simulink library "ddm"  (R2021b)
settings: Solver=VariableStepAuto  StartTime=0.0  StopTime=10.0  RelTol=1e-3
undefined symbols (not defined in the file): ADDM_FrTMTqDev_X_Nm, ADDM_RrTMTqDev_X_Nm, ENUM_ADASACCSTA_ERROR, ENUM_ADASACCSTA_OFF, ENUM_ADASACCSTA_STANDBY, ENUM_ALLOWMOV_ALLOWREADY, ENUM_APS, ENUM_BRKSTA_ERROR, ENUM_BRKSTA_OFF, ENUM_BRKSTA_ON, ENUM_BRKSW_INVALID, ENUM_BRKSW_OFF, ENUM_BRKSW_ON, ENUM_CHGPREACTERRSTA_OBCPRE, ENUM_DCDCFAULTSTA_ANYFAULTLV1, ENUM_DCDCFAULTSTA_ANYFAULTLV2, ENUM_DRIVETRAIN_AWD, ENUM_DRIVETRAIN_FWD, ENUM_DRIVETRAIN_RWD, ENUM_EDUDRTSTA_NORMAL, ENUM_EPBERROR_FAILED, ENUM_EPBSTA_APPLIED, ENUM_EPBSTA_RELEASED, ENUM_ESCAPSSta_APSUNAVAILABLE, ENUM_GEARACTUALPOSN_INVALID, ENUM_GEARACTUALPOSN_P, ENUM_HVBATTREADYPRE_READY, ENUM_HWRESETSTA_HWRESETING, ENUM_MCUWARN_LV0, ENUM_MCUWARN_LV1, ENUM_MCUWARN_LV2, ENUM_MCUWARN_LV3, ENUM_MCUWARN_NOERROR, ENUM_OBCFAULTSTA_ANYFAULT, ENUM_PAS_R2F2, ENUM_PDFAULT_BATTPDFAIL, ENUM_PDFAULT_DCDCDISABLE, ENUM_PDFAULT_MCUDISABLE, ENUM_PDFAULT_MCUDISCHRG, ENUM_POWERSTA_OFF, ENUM_POWERSTA_ON, ENUM_POWERSTA_READY, ENUM_POWERSTA_STANDBY, ENUM_PRESSINDI_LOW, ENUM_PUFAULT_BATTUPFAIL, ENUM_PUFAULT_DCDCENABLEFAIL, ENUM_PUFAULT_PRECHRGCHKFAIL, ENUM_PUFAULT_SAFETYCHKFAIL, ENUM_PWRSTASW_OFF, ENUM_PWRSTASW_OFFA, ENUM_PWRSTASW_OFFCHVCHRG, ENUM_PWRSTASW_OFFCLVCHRG, ENUM_PWRSTASW_ON, ENUM_PWRSTASW_ONHVCHRG, ENUM_PWRSTASW_READY, ENUM_PWRSTASW_STANDBY, ENUM_RAPSErrWarnSta_NORMAL, ENUM_RAPSErrWarnSta_RAPSERRLV1, ENUM_SHIFTCOMMAND_P, ENUM_SHIFTERERRSTA_PBUTTONFAILURE ... (+471)
libraries: hcu_lib x540, simulink x3
(part 9 of 26)

== system ddm/DDM/DDM/PMM/Fault level ==
  task_time_s : Inport
  VPMM_PwrStaSW_enum : Inport  Port=2
  VPMM_PowerSta_enum : Inport  Port=3
  VINP_BMSWarn1_flg : Inport  Port=4
  VINP_BMSWarn2_flg : Inport  Port=5
  VINP_BMSWarn3_flg : Inport  Port=6
  VINP_BMSWarn4_flg : Inport  Port=7
  VINP_BMSWarn5_flg : Inport  Port=8
  VINP_BMSWarn6_flg : Inport  Port=9
  VINP_BMSWarn7_flg : Inport  Port=10
  VINP_BMSWarn8_flg : Inport  Port=11
  VINP_DCDCFaultSta_enum : Inport  Port=12
  VPMM_DrivetrainSelect_enum : Inport  Port=13
  VDDM_C3BMS6LCCFS_flg : Inport  Port=14
  VDDM_C3CCU2LCCFS_flg : Inport  Port=15
  VDDM_MCUF1NoComCFS_flg : Inport  Port=16
  VDDM_MCUR1NoComCFS_flg : Inport  Port=17
  VDDM_MCUWarnF_enum : Inport  Port=18
  VDDM_MCUWarnR_enum : Inport  Port=19
  VINP_OBCFaultSta_enum : Inport  Port=20
  DTC_clear_request : Inport  Port=21
  No_CAN3_BUS_OFF : Inport  Port=22
  VDDM_C3CCU2RCCFS_flg : Inport  Port=23
  VDDM_C3CCU2CSCFS_flg : Inport  Port=24
  VDDM_MCUR1RCErrCFS_flg : Inport  Port=25
  VDDM_MCUR1CSErrCFS_flg : Inport  Port=26
  VDDM_MCUF1RCErrCFS_flg : Inport  Port=27
  VDDM_MCUF1CSErrCFS_flg : Inport  Port=28
  VDDM_C3BMS6RCCFS_flg : Inport  Port=29
  VDDM_C3BMS6CSCFS_flg : Inport  Port=30
  No_CAN1_BUS_OFF : Inport  Port=31
  VDDM_ESC1SigErr_flg : Inport  Port=32
  VDDM_ESC5SigErr_flg : Inport  Port=33
  ZoneFrMalfunLevel_enum : Inport  Port=34
  VDDM_FrVCUNoComCFS_flg : Inport  Port=35
  VINP_ShifterFailsta_enum : Inport  Port=36
  VDDM_Shifter1NoComCFS_flg : Inport  Port=37
  VDDM_Shifter1RCErrCFS_flg : Inport  Port=38
  VDDM_Shifter1CSErrCFS_flg : Inport  Port=39
  VINP_ZoneDrMalfunLevel_enum : Inport  Port=40
  No_CAN4_BUS_OFF : Inport  Port=41
  VDDM_DrVCUNoComCFS_flg : Inport  Port=42
  Fault level 1 subsystem error : Subsystem
  Fault level 2 subsystem error : Subsystem
  Fault level 3 subsystem error : Subsystem
  Fault level 4 subsystem error1 : Subsystem
  VDDM_Lv1ErrDTC_raw32 : Outport
  VDDM_Lv2ErrDTC_raw32 : Outport  Port=2
  VDDM_Lv3ErrDTC_raw32 : Outport  Port=3
  VDDM_Lv4ErrDTC_raw32 : Outport  Port=4
  VDDM_Lv1ErrCFS_flg : Outport  Port=5
  VDDM_Lv2ErrCFS_flg : Outport  Port=6
  VDDM_Lv3ErrCFS_flg : Outport  Port=7
  VDDM_Lv4ErrCFS_flg : Outport  Port=8
  VDDM_EDriveSysErrFaultLv1_flg : Outport  Port=9
  wires:
  [No_CAN3_BUS_OFF] -> Fault level 4 subsystem error1/8(No_CAN3_BUS_OFF)
  [DTC_clear_request] -> Fault level 4 subsystem error1/7(DTC_clear_request)
  [DTC_clear_request] -> Fault level 3 subsystem error/11(DTC_clear_request)
  [No_CAN3_BUS_OFF] -> Fault level 3 subsystem error/12(No_CAN3_BUS_OFF)
  [No_CAN3_BUS_OFF] -> Fault level 2 subsystem error/15(No_CAN3_BUS_OFF)
  [DTC_clear_request] -> Fault level 2 subsystem error/14(DTC_clear_request)
  [DTC_clear_request] -> Fault level 1 subsystem error/16(DTC_clear_request)
  [No_CAN3_BUS_OFF] -> Fault level 1 subsystem error/17(No_CAN3_BUS_OFF)
  DTC_clear_request/1 -> [DTC_clear_request]
  No_CAN3_BUS_OFF/1 -> [No_CAN3_BUS_OFF]
  [VDDM_MCUWarnR_enum] -> Fault level 1 subsystem error/13(VDDM_MCUWarnR_enum)
  [VDDM_MCUWarnF_enum] -> Fault level 1 subsystem error/12(VDDM_MCUWarnF_enum)
  [VDDM_MCUWarnF_enum] -> Fault level 3 subsystem error/8(VDDM_MCUWarnF_enum)
  [VDDM_MCUWarnR_enum] -> Fault level 3 subsystem error/9(VDDM_MCUWarnR_enum)
  [VPMM_DrivetrainSelect_enum] -> Fault level 3 subsystem error/10(VPMM_DrivetrainSelect_enum)
  [VDDM_MCUWarnR_enum] -> Fault level 2 subsystem error/12(VDDM_MCUWarnR_enum)
  [VDDM_MCUWarnF_enum] -> Fault level 2 subsystem error/11(VDDM_MCUWarnF_enum)
  [VPMM_DrivetrainSelect_enum] -> Fault level 2 subsystem error/13(VPMM_DrivetrainSelect_enum)
  [VINP_OBCFaultSta_enum] -> Fault level 1 subsystem error/14(VINP_OBCFaultSta_enum)
  VINP_OBCFaultSta_enum/1 -> [VINP_OBCFaultSta_enum]
  VDDM_MCUWarnR_enum/1 -> [VDDM_MCUWarnR_enum]
  VDDM_MCUWarnF_enum/1 -> [VDDM_MCUWarnF_enum]
  [VDDM_C3CCU2LCCFS_flg] -> Fault level 2 subsystem error/5(VDDM_C3CCU2LCCFS_flg)
  [VDDM_C3CCU2LCCFS_flg] -> Fault level 1 subsystem error/5(VDDM_C3CCU2LCCFS_flg)
  VDDM_C3CCU2LCCFS_flg/1 -> [VDDM_C3CCU2LCCFS_flg]
  [VDDM_C3BMS6LCCFS_flg] -> Fault level 4 subsystem error1/4(VDDM_C3BMS6LCCFS_flg)
  [VDDM_C3BMS6LCCFS_flg] -> Fault level 3 subsystem error/4(VDDM_C3BMS6LCCFS_flg)
  [VDDM_MCUR1NoComCFS_flg] -> Fault level 3 subsystem error/6(VDDM_MCUR1NoComCFS_flg)
  [VDDM_MCUF1NoComCFS_flg] -> Fault level 3 subsystem error/5(VDDM_MCUF1NoComCFS_flg)
  [VDDM_MCUF1NoComCFS_flg] -> Fault level 2 subsystem error/6(VDDM_MCUF1NoComCFS_flg)
  [VDDM_MCUR1NoComCFS_flg] -> Fault level 2 subsystem error/7(VDDM_MCUR1NoComCFS_flg)
  [VDDM_MCUF1NoComCFS_flg] -> Fault level 1 subsystem error/6(VDDM_MCUF1NoComCFS_flg)
  [VDDM_MCUR1NoComCFS_flg] -> Fault level 1 subsystem error/7(VDDM_MCUR1NoComCFS_flg)
  VDDM_MCUF1NoComCFS_flg/1 -> [VDDM_MCUF1NoComCFS_flg]
  VDDM_MCUR1NoComCFS_flg/1 -> [VDDM_MCUR1NoComCFS_flg]
  [VDDM_C3BMS6LCCFS_flg] -> Fault level 2 subsystem error/4(VDDM_C3BMS6LCCFS_flg)
  [VDDM_C3BMS6LCCFS_flg] -> Fault level 1 subsystem error/4(VDDM_C3BMS6LCCFS_flg)
  VDDM_C3BMS6LCCFS_flg/1 -> [VDDM_C3BMS6LCCFS_flg]
  [task_time_s] -> Fault level 4 subsystem error1/1(task_time_s)
  [VPMM_DrivetrainSelect_enum] -> Fault level 1 subsystem error/15(VPMM_DrivetrainSelect_enum)
  VPMM_DrivetrainSelect_enum/1 -> [VPMM_DrivetrainSelect_enum]
  [VPMM_PowerSta_enum] -> Fault level 3 subsystem error/2(VPMM_PowerSta_enum)
  [VPMM_PwrStaSW_enum] -> Fault level 3 subsystem error/3(VPMM_PwrStaSW_enum)
  [task_time_s] -> Fault level 3 subsystem error/1(task_time_s)
  [VINP_DCDCFaultSta_enum] -> Fault level 1 subsystem error/11(VINP_DCDCFaultSta_enum)
  [VINP_DCDCFaultSta_enum] -> Fault level 2 subsystem error/10(VINP_DCDCFaultSta_enum)
  VINP_DCDCFaultSta_enum/1 -> [VINP_DCDCFaultSta_enum]
  [task_time_s] -> Fault level 2 subsystem error/1(task_time_s)
  [VPMM_PwrStaSW_enum] -> Fault level 2 subsystem error/3(VPMM_PwrStaSW_enum)
  [VPMM_PowerSta_enum] -> Fault level 2 subsystem error/2(VPMM_PowerSta_enum)
  [VPMM_PowerSta_enum] -> Fault level 1 subsystem error/2(VPMM_PowerSta_enum)
  [VPMM_PwrStaSW_enum] -> Fault level 1 subsystem error/3(VPMM_PwrStaSW_enum)
  [task_time_s] -> Fault level 1 subsystem error/1(task_time_s)
  VPMM_PowerSta_enum/1 -> [VPMM_PowerSta_enum]
  VPMM_PwrStaSW_enum/1 -> [VPMM_PwrStaSW_enum]
  task_time_s/1 -> [task_time_s]
  [VDDM_C3CCU2RCCFS_flg] -> Fault level 1 subsystem error/18(VDDM_C3CCU2RCCFS_flg)
  [VDDM_C3CCU2CSCFS_flg] -> Fault level 1 subsystem error/19(VDDM_C3CCU2CSCFS_flg)
  [VDDM_MCUR1RCErrCFS_flg] -> Fault level 1 subsystem error/20(VDDM_MCUR1RCErrCFS_flg)
  [VDDM_MCUR1CSErrCFS_flg] -> Fault level 1 subsystem error/21(VDDM_MCUR1CSErrCFS_flg)
  [VDDM_MCUF1RCErrCFS_flg] -> Fault level 1 subsystem error/22(VDDM_MCUF1RCErrCFS_flg)
  [VDDM_MCUF1CSErrCFS_flg] -> Fault level 1 subsystem error/23(VDDM_MCUF1CSErrCFS_flg)
  [VDDM_C3BMS6RCCFS_flg] -> Fault level 1 subsystem error/24(VDDM_C3BMS6RCCFS_flg)
  [VDDM_C3BMS6CSCFS_flg] -> Fault level 1 subsystem error/25(VDDM_C3BMS6CSCFS_flg)
  [No_CAN1_BUS_OFF] -> Fault level 1 subsystem error/26(No_CAN1_BUS_OFF)
  [VDDM_ESC1SigErr_flg] -> Fault level 1 subsystem error/27(VDDM_ESC1SigErr_flg)
  [VDDM_ESC5SigErr_flg] -> Fault level 1 subsystem error/28(VDDM_ESC5SigErr_flg)
  [VINP_ShifterFailsta_enum] -> Fault level 1 subsystem error/29(VINP_ShifterFailsta_enum)
  [VDDM_Shifter1NoComCFS_flg] -> Fault level 1 subsystem error/30(VDDM_Shifter1NoComCFS_flg)
  [VDDM_Shifter1RCErrCFS_flg] -> Fault level 1 subsystem error/31(VDDM_Shifter1RCErrCFS_flg)
  [VDDM_Shifter1CSErrCFS_flg] -> Fault level 1 subsystem error/32(VDDM_Shifter1CSErrCFS_flg)
  [VINP_ZoneDrMalfunLevel_enum] -> Fault level 1 subsystem error/33(VINP_ZoneDrMalfunLevel_enum)
  [No_CAN4_BUS_OFF] -> Fault level 1 subsystem error/34(No_CAN4_BUS_OFF)
  [VDDM_DrVCUNoComCFS_flg] -> Fault level 1 subsystem error/35(VDDM_DrVCUNoComCFS_flg)
  [ZoneFrMalfunLevel_enum] -> Fault level 1 subsystem error/36(ZoneFrMalfunLevel_enum)
  [VDDM_FrVCUNoComCFS_flg] -> Fault level 1 subsystem error/37(VDDM_FrVCUNoComCFS_flg)
  [VDDM_C3CCU2RCCFS_flg] -> Fault level 2 subsystem error/16(VDDM_C3CCU2RCCFS_flg)
  [VDDM_C3CCU2CSCFS_flg] -> Fault level 2 subsystem error/17(VDDM_C3CCU2CSCFS_flg)
  [VDDM_MCUR1RCErrCFS_flg] -> Fault level 2 subsystem error/18(VDDM_MCUR1RCErrCFS_flg)
  [VDDM_MCUR1CSErrCFS_flg] -> Fault level 2 subsystem error/19(VDDM_MCUR1CSErrCFS_flg)
  [VDDM_MCUF1RCErrCFS_flg] -> Fault level 2 subsystem error/20(VDDM_MCUF1RCErrCFS_flg)
  [VDDM_MCUF1CSErrCFS_flg] -> Fault level 2 subsystem error/21(VDDM_MCUF1CSErrCFS_flg)
  [VDDM_C3BMS6RCCFS_flg] -> Fault level 2 subsystem error/22(VDDM_C3BMS6RCCFS_flg)
  [VDDM_C3BMS6CSCFS_flg] -> Fault level 2 subsystem error/23(VDDM_C3BMS6CSCFS_flg)
  [VINP_ZoneDrMalfunLevel_enum] -> Fault level 2 subsystem error/24(ZoneDrMalfunLevel_enum)
  [No_CAN4_BUS_OFF] -> Fault level 2 subsystem error/25(No_CAN4_BUS_OFF)
  [VDDM_DrVCUNoComCFS_flg] -> Fault level 2 subsystem error/26(VDDM_DrVCUNoComCFS_flg)
  [ZoneFrMalfunLevel_enum] -> Fault level 2 subsystem error/27(ZoneFrMalfunLevel_enum)
  [VDDM_FrVCUNoComCFS_flg] -> Fault level 2 subsystem error/28(VDDM_FrVCUNoComCFS_flg)
  [VDDM_MCUR1RCErrCFS_flg] -> Fault level 3 subsystem error/13(VDDM_MCUR1RCErrCFS_flg)
  [VDDM_MCUR1CSErrCFS_flg] -> Fault level 3 subsystem error/14(VDDM_MCUR1CSErrCFS_flg)
  [VDDM_MCUF1RCErrCFS_flg] -> Fault level 3 subsystem error/15(VDDM_MCUF1RCErrCFS_flg)
  [VDDM_MCUF1CSErrCFS_flg] -> Fault level 3 subsystem error/16(VDDM_MCUF1CSErrCFS_flg)
  [VDDM_C3BMS6RCCFS_flg] -> Fault level 3 subsystem error/17(VDDM_C3BMS6RCCFS_flg)
  [VDDM_C3BMS6CSCFS_flg] -> Fault level 3 subsystem error/18(VDDM_C3BMS6CSCFS_flg)
  [VINP_ZoneDrMalfunLevel_enum] -> Fault level 3 subsystem error/19(ZoneDrMalfunLevel_enum)
  [No_CAN4_BUS_OFF] -> Fault level 3 subsystem error/20(No_CAN4_BUS_OFF)
  [VDDM_DrVCUNoComCFS_flg] -> Fault level 3 subsystem error/21(VDDM_DrVCUNoComCFS_flg)
  [ZoneFrMalfunLevel_enum] -> Fault level 3 subsystem error/22(ZoneFrMalfunLevel_enum)
  [VDDM_FrVCUNoComCFS_flg] -> Fault level 3 subsystem error/23(VDDM_FrVCUNoComCFS_flg)
  [VPMM_PwrStaSW_enum] -> Fault level 4 subsystem error1/3(VPMM_PwrStaSW_enum)
  [VPMM_PowerSta_enum] -> Fault level 4 subsystem error1/2(VPMM_PowerSta_enum)
  [VDDM_C3BMS6RCCFS_flg] -> Fault level 4 subsystem error1/9(VDDM_C3BMS6RCCFS_flg)
  [VDDM_C3BMS6CSCFS_flg] -> Fault level 4 subsystem error1/10(VDDM_C3BMS6CSCFS_flg)
  [VINP_ZoneDrMalfunLevel_enum] -> Fault level 4 subsystem error1/11(ZoneDrMalfunLevel_enum)
  [No_CAN4_BUS_OFF] -> Fault level 4 subsystem error1/12(No_CAN4_BUS_OFF)
  [VDDM_DrVCUNoComCFS_flg] -> Fault level 4 subsystem error1/13(VDDM_DrVCUNoComCFS_flg)
  [ZoneFrMalfunLevel_enum] -> Fault level 4 subsystem error1/14(ZoneFrMalfunLevel_enum)
  [VDDM_FrVCUNoComCFS_flg] -> Fault level 4 subsystem error1/15(VDDM_FrVCUNoComCFS_flg)
  VINP_BMSWarn1_flg/1 -> [VINP_BMSWarn1_flg]
  VINP_BMSWarn2_flg/1 -> [VINP_BMSWarn2_flg]
  VINP_BMSWarn3_flg/1 -> [VINP_BMSWarn3_flg]
  VINP_BMSWarn4_flg/1 -> [VINP_BMSWarn4_flg]
  VINP_BMSWarn5_flg/1 -> [VINP_BMSWarn5_flg]
  VINP_BMSWarn6_flg/1 -> [VINP_BMSWarn6_flg]
  VINP_BMSWarn7_flg/1 -> [VINP_BMSWarn7_flg]
  VINP_BMSWarn8_flg/1 -> [VINP_BMSWarn8_flg]
  [VINP_BMSWarn1_flg] -> Fault level 1 subsystem error/8(VINP_BMSWarn1_flg)
  [VINP_BMSWarn2_flg] -> Fault level 1 subsystem error/9(VINP_BMSWarn2_flg)
  [VINP_BMSWarn3_flg] -> Fault level 1 subsystem error/10(VINP_BMSWarn3_flg)
  [VINP_BMSWarn4_flg] -> Fault level 2 subsystem error/8(VINP_BMSWarn4_flg)
  [VINP_BMSWarn5_flg] -> Fault level 2 subsystem error/9(VINP_BMSWarn5_flg)
  [VINP_BMSWarn6_flg] -> Fault level 3 subsystem error/7(VINP_BMSWarn6_flg)
  [VINP_BMSWarn7_flg] -> Fault level 4 subsystem error1/5(VINP_BMSWarn7_flg)
  [VINP_BMSWarn8_flg] -> Fault level 4 subsystem error1/6(VINP_BMSWarn8_flg)
  Fault level 1 subsystem error/1(VDDM_Lv1ErrCFS_flg) -> [VDDM_Lv1ErrCFS_flg]
  Fault level 1 subsystem error/2(VDDM_Lv1ErrDTC_raw32) -> [VDDM_Lv1ErrDTC_raw32]
  Fault level 2 subsystem error/1(VDDM_Lv2ErrCFS_flg) -> [VDDM_Lv2ErrCFS_flg]
  Fault level 3 subsystem error/1(VDDM_Lv3ErrCFS_flg) -> [VDDM_Lv3ErrCFS_flg]
  Fault level 4 subsystem error1/1(VDDM_Lv4ErrCFS_flg) -> [VDDM_Lv4ErrCFS_flg]
  Fault level 2 subsystem error/2(VDDM_Lv2ErrDTC_raw32) -> [VDDM_Lv2ErrDTC_raw32]
  Fault level 3 subsystem error/2(VDDM_Lv3ErrDTC_raw32) -> [VDDM_Lv3ErrDTC_raw32]
  Fault level 4 subsystem error1/2(VDDM_Lv4ErrDTC_raw32) -> [VDDM_Lv4ErrDTC_raw32]
  [VDDM_Lv1ErrDTC_raw32] -> VDDM_Lv1ErrDTC_raw32/1
  [VDDM_Lv2ErrDTC_raw32] -> VDDM_Lv2ErrDTC_raw32/1
  [VDDM_Lv3ErrDTC_raw32] -> VDDM_Lv3ErrDTC_raw32/1
  [VDDM_Lv4ErrDTC_raw32] -> VDDM_Lv4ErrDTC_raw32/1
  [VDDM_Lv1ErrCFS_flg] -> VDDM_Lv1ErrCFS_flg/1
  [VDDM_Lv2ErrCFS_flg] -> VDDM_Lv2ErrCFS_flg/1
  [VDDM_Lv3ErrCFS_flg] -> VDDM_Lv3ErrCFS_flg/1
  [VDDM_Lv4ErrCFS_flg] -> VDDM_Lv4ErrCFS_flg/1
  VDDM_MCUF1RCErrCFS_flg/1 -> [VDDM_MCUF1RCErrCFS_flg]
  VDDM_C3BMS6RCCFS_flg/1 -> [VDDM_C3BMS6RCCFS_flg]
  VDDM_MCUR1RCErrCFS_flg/1 -> [VDDM_MCUR1RCErrCFS_flg]
  VDDM_MCUR1CSErrCFS_flg/1 -> [VDDM_MCUR1CSErrCFS_flg]
  VDDM_C3CCU2CSCFS_flg/1 -> [VDDM_C3CCU2CSCFS_flg]
  VDDM_C3CCU2RCCFS_flg/1 -> [VDDM_C3CCU2RCCFS_flg]
  VDDM_MCUF1CSErrCFS_flg/1 -> [VDDM_MCUF1CSErrCFS_flg]
  VDDM_ESC5SigErr_flg/1 -> [VDDM_ESC5SigErr_flg]
  VDDM_ESC1SigErr_flg/1 -> [VDDM_ESC1SigErr_flg]
  No_CAN1_BUS_OFF/1 -> [No_CAN1_BUS_OFF]
  VDDM_C3BMS6CSCFS_flg/1 -> [VDDM_C3BMS6CSCFS_flg]
  ZoneFrMalfunLevel_enum/1 -> [ZoneFrMalfunLevel_enum]
  VDDM_FrVCUNoComCFS_flg/1 -> [VDDM_FrVCUNoComCFS_flg]
  No_CAN4_BUS_OFF/1 -> [No_CAN4_BUS_OFF]
  VINP_ZoneDrMalfunLevel_enum/1 -> [VINP_ZoneDrMalfunLevel_enum]
  VDDM_DrVCUNoComCFS_flg/1 -> [VDDM_DrVCUNoComCFS_flg]
  VDDM_Shifter1NoComCFS_flg/1 -> [VDDM_Shifter1NoComCFS_flg]
  VDDM_Shifter1RCErrCFS_flg/1 -> [VDDM_Shifter1RCErrCFS_flg]
  VINP_ShifterFailsta_enum/1 -> [VINP_ShifterFailsta_enum]
  VDDM_Shifter1CSErrCFS_flg/1 -> [VDDM_Shifter1CSErrCFS_flg]
  Fault level 1 subsystem error/3(VDDM_EDriveSysErrFaultLv1_flg) -> [VDDM_EDriveSysErrFaultLv1_flg]
  [VDDM_EDriveSysErrFaultLv1_flg] -> VDDM_EDriveSysErrFaultLv1_flg/1

== system ddm/DDM/DDM/PMM/Key authentication failed ==
  note: Diagnostics and Fault Handling
  note: Test Pass Criteria
  note: Release Condition After Decision
  note: Test Detection Criteria
  task_time_s : Inport
  VPMM_PowerSta_enum : Inport  Port=2
  VPMM_PwrStaSW_enum : Inport  Port=3
  DTC_clear_request : Inport  Port=4
  VDKC_DKCAuthSta_enum : Inport  Port=5
  VINP_CANMsgValidDKC2_flg : Inport  Port=6
  VINP_CANMsgValidDKC1_flg : Inport  Port=7
  VDDM_ClearZevDTCcmd_flg : Inport  Port=8
  Constant1 : Constant  Value=TRUE
  Constant10 : Constant  Value=ENUM_POWERSTA_STANDBY
  Constant12 : Constant  Value=FALSE
  Constant13 : Constant  Value=KDDM_KeyAuthDTC_cnt
  Constant14 : Constant  Value=KDDM_KeyAuthPassTO_s
  Constant17 : Constant  Value=KDDM_KeyAuthPassTO_s
  Constant18 : Constant  Value=KDDM_KeyAuthDTC_cnt
  Constant2 : Constant  Value=ENUM_PWRSTASW_OFF
  Constant22 : Constant  Value=FALSE
  Constant28 : Constant  Value=ENUM_PWRSTASW_OFF
  Constant30 : Constant  Value=KDDM_KeyAuthDiagnosisOffSW_flg
  Constant31 : Constant  Value=ENUM_POWERSTA_OFF
  Constant6 : Constant  Value=ZERO_INT
  Constant9 : Constant  Value=KDDM_KeyAuthDetTO_s
  DTC_Couter1 : hcu_lib/Basic_Blocks/DTC_Couter
  DTC_Info : hcu_lib/Basic_Blocks/DTC_Info
  Equal1 : RelationalOperator  Operator=~=  OutDataTypeStr=boolean  RndMeth=Simplest
  Equal10 : RelationalOperator  Operator===  OutDataTypeStr=boolean  RndMeth=Simplest
  Equal2 : RelationalOperator  Operator=~=  OutDataTypeStr=boolean  RndMeth=Simplest
  Equal8 : RelationalOperator  OutDataTypeStr=boolean  RndMeth=Simplest
  Equal9 : RelationalOperator  Operator===  OutDataTypeStr=boolean  RndMeth=Simplest
  Logical Operator : Logic  Inputs=3  AllPortsSameDT=off  OutDataTypeStr=boolean
  Logical Operator1 : Logic  Inputs=3  AllPortsSameDT=off  OutDataTypeStr=boolean
  Logical Operator16 : Logic  Operator=OR  Inputs=4  AllPortsSameDT=off  OutDataTypeStr=boolean
  Logical Operator17 : Logic  AllPortsSameDT=off  OutDataTypeStr=boolean
  Logical Operator21 : Logic  Operator=NOT  AllPortsSameDT=off  OutDataTypeStr=boolean
  Relational Operator1 : RelationalOperator  Operator=>  OutDataTypeStr=boolean  RndMeth=Simplest
  Switch1 : Switch  Criteria=u2 ~= 0
  Switch8 : Switch  Criteria=u2 ~= 0
  Switch9 : Switch  Criteria=u2 ~= 0
  Terminator : Terminator
  Test Detection Criteria1 : hcu_lib/Basic_Blocks/Test Detection Criteria
  Timer2 : hcu_lib/Basic_Blocks/Timer
  Unit Delay1 : UnitDelay  SampleTime=-1  HasFrameUpgradeWarning=on
  VDDM_KeyAuthDTC_raw32 : Outport
  VDDM_KeyAuthCFS_flg : Outport  Port=2
  wires:
  [VDDM_KeyAuthCFS_flg] -> VDDM_KeyAuthCFS_flg/1
  [VDDM_KeyAuthPass_flg] -> Logical Operator16/3
  [VPMM_PwrStaSW_enum] -> Equal1/1
  Constant28/1 -> Equal1/2
  Test Detection Criteria1/1 -> [VDDM_KeyAuthDet_flg]  "VDDM_KeyAuthDet_flg"
  [VDKC_DKCAuthSta_enum] -> Switch8/1
  Equal9/1 -> Logical Operator17/1
  Constant10/1 -> Equal10/2
  Constant17/1 -> Equal8/2
  Constant14/1 -> Timer2/4
  Constant22/1 -> Switch9/1
  [VPMM_PowerSta_enum] -> Equal10/1
  [VDDM_KeyAuthCFSRls_flg] -> DTC_Couter1/2
  Constant18/1 -> DTC_Couter1/3
  DTC_Couter1/1 -> [VDDM_KeyAuthCFS_flg]  "VDDM_KeyAuthCFS_flg"
  Relational Operator1/1 -> Terminator/1  "VDDM_KeyAuthDFS_flg"
  Timer2/1 -> Equal8/1
  Switch9/1 -> Test Detection Criteria1/1
  Constant12/1 -> Switch1/3
  Logical Operator21/1 -> Timer2/1
  Equal10/1 -> Logical Operator17/2
  DTC_Couter1/2 -> Relational Operator1/1  "VDDM_KeyAuthDTC_cnt"
  Constant31/1 -> Equal9/2
  Logical Operator17/1 -> Logical Operator16/1
  [VDDM_ClearZevDTCcmd_flg] -> Logical Operator16/2
  [task_time_s] -> Timer2/3
  Constant30/1 -> Logical Operator16/4
  Constant1/1 -> Switch8/3
  [VDDM_KeyAuthCFSRls_flg] -> Switch9/2
  Switch1/1 -> Switch9/3
  [task_time_s] -> Test Detection Criteria1/2
  [VPMM_PowerSta_enum] -> Unit Delay1/1
  Switch8/1 -> Logical Operator21/1, Timer2/2
  Equal8/1 -> [VDDM_KeyAuthPass_flg]  "VDDM_KeyAuthPass_flg"
  Constant6/1 -> Relational Operator1/2
  Unit Delay1/1 -> Equal9/1
  Constant9/1 -> Test Detection Criteria1/4
  [VDDM_KeyAuthDet_flg] -> DTC_Couter1/1
  Logical Operator16/1 -> [VDDM_KeyAuthCFSRls_flg]  "VDDM_KeyAuthCFSRls_flg"
  Constant13/1 -> Test Detection Criteria1/3
  VPMM_PowerSta_enum/1 -> [VPMM_PowerSta_enum]
  VPMM_PwrStaSW_enum/1 -> [VPMM_PwrStaSW_enum]
  task_time_s/1 -> [task_time_s]
  VDKC_DKCAuthSta_enum/1 -> [VDKC_DKCAuthSta_enum]
  DTC_clear_request/1 -> [DTC_clear_request]
  [VDDM_KeyAuthPass_flg] -> DTC_Info/2
  [VDDM_KeyAuthCFS_flg] -> DTC_Info/3
  DTC_Info/1 -> VDDM_KeyAuthDTC_raw32/1  "VDDM_KeyAuthDTC_raw32"
  [VDDM_KeyAuthDet_flg] -> DTC_Info/1
  [VDDM_ClearZevDTCcmd_flg] -> DTC_Info/4
  [VDKC_DKCAuthSta_enum] -> Switch1/1
  VINP_CANMsgValidDKC2_flg/1 -> [VINP_CANMsgValidDKC2_flg]
  VINP_CANMsgValidDKC1_flg/1 -> [VINP_CANMsgValidDKC1_flg]
  Logical Operator/1 -> Switch1/2
  Equal1/1 -> Logical Operator/1
  [VINP_CANMsgValidDKC1_flg] -> Logical Operator/2
  [VINP_CANMsgValidDKC2_flg] -> Logical Operator/3
  [VINP_CANMsgValidDKC1_flg] -> Logical Operator1/2
  Equal2/1 -> Logical Operator1/1
  [VPMM_PwrStaSW_enum] -> Equal2/1
  Logical Operator1/1 -> Switch8/2
  Constant2/1 -> Equal2/2
  [VINP_CANMsgValidDKC2_flg] -> Logical Operator1/3
  VDDM_ClearZevDTCcmd_flg/1 -> [VDDM_ClearZevDTCcmd_flg]

== system ddm/DDM/DDM/PMM/LV ==
  task_time_s : Inport
  VPMM_PwrStaSW_enum : Inport  Port=2
  VPMM_PowerSta_enum : Inport  Port=3
  VINP_LVBattDet12V_V : Inport  Port=4
  VINP_CANMsgValidBMS5_flg : Inport  Port=5
  DTC_clear_request : Inport  Port=6
  VDDM_AuxBattVolV_V : Inport  Port=7
  VDDM_ClearZevDTCcmd_flg : Inport  Port=8
  VINP_VehicleType_enum : Inport  Port=9
  Constant1 : Constant  Value=ENUM_VEHICLETYPE_D31L24
  Constant2 : Constant  Value=TRUE
  Constant7 : Constant  Value=ENUM_VEHICLETYPE_D31L24
  Initial LV battery voltage too low : Subsystem
  LV analog input error : Subsystem
  LV power supply voltage too high : Subsystem
  LV power supply voltage too low : Subsystem
  Logical Operator : Logic  Operator=OR  Inputs=4  AllPortsSameDT=off  OutDataTypeStr=boolean
  Logical Operator1 : Logic  Operator=OR  AllPortsSameDT=off  OutDataTypeStr=boolean
  Relational Operator1 : RelationalOperator  Operator=~=  OutDataTypeStr=boolean  RndMeth=Simplest
  Relational Operator5 : RelationalOperator  Operator=~=  OutDataTypeStr=boolean  RndMeth=Simplest
  Switch : Switch  Criteria=u2 ~= 0
  Switch2 : Switch  Criteria=u2 ~= 0
  VDDM_IniLVLoDTC_raw32 : Outport
  VDDM_LVSupLoDTC_raw32 : Outport  Port=2
  VDDM_LVSupHiDTC_raw32 : Outport  Port=3
  VDDM_LVInErrDTC_raw32 : Outport  Port=4
  VDDM_IniLVLoCFS_flg : Outport  Port=5
  VDDM_LVSupLoCFS_flg : Outport  Port=6
  VDDM_LVSupHiCFS_flg : Outport  Port=7
  VDDM_LVInErrCFS_flg : Outport  Port=8
  VDDM_PMMBattErr_flg : Outport  Port=9
  VDDM_EDriveSysErrLVSup_flg : Outport  Port=10
  wires:
  DTC_clear_request/1 -> [DTC_clear_request]
  [VDDM_ClearZevDTCcmd_flg] -> LV power supply voltage too high/6(DTC_clear_request)
  [VDDM_AuxBatVolt_V] -> LV power supply voltage too high/4(VDDM_AuxBatVolt_V)
  [VPMM_PowerSta_enum] -> LV power supply voltage too high/2(VPMM_PowerSta_enum)
  [VINP_CANMsgValidBMS5_flg] -> LV power supply voltage too high/5(VINP_CANMsgValidBMS5_flg)
  [VPMM_PwrStaSW_enum] -> LV power supply voltage too high/3(VPMM_PwrStaSW_enum)
  [task_time_s] -> LV power supply voltage too high/1(task_time_s)
  [VDDM_AuxBatVolt_V] -> LV power supply voltage too low/4(VDDM_AuxBatVolt_V)
  [VINP_CANMsgValidBMS5_flg] -> LV power supply voltage too low/5(VINP_CANMsgValidBMS5_flg)
  [task_time_s] -> LV power supply voltage too low/1(task_time_s)
  [VDDM_ClearZevDTCcmd_flg] -> LV power supply voltage too low/6(DTC_clear_request)
  [VPMM_PwrStaSW_enum] -> LV power supply voltage too low/3(VPMM_PwrStaSW_enum)
  [VPMM_PowerSta_enum] -> LV power supply voltage too low/2(VPMM_PowerSta_enum)
  VINP_LVBattDet12V_V/1 -> [VINP_LVBattDet12V_V]
  task_time_s/1 -> [task_time_s]
  VPMM_PwrStaSW_enum/1 -> [VPMM_PwrStaSW_enum]
  VPMM_PowerSta_enum/1 -> [VPMM_PowerSta_enum]
  LV power supply voltage too low/1(VDDM_LVSupLoDTC_raw32) -> VDDM_LVSupLoDTC_raw32/1  "VDDM_LVSupLoDTC_raw32"
  LV power supply voltage too high/1(VDDM_LVSupHiDTC_raw32) -> VDDM_LVSupHiDTC_raw32/1  "VDDM_LVSupHiDTC_raw32"
  LV power supply voltage too low/2(VDDM_LVSupLoCFS_flg) -> [VDDM_LVSupLoCFS_flg]
  LV power supply voltage too high/2(VDDM_LVSupHiCFS_flg) -> [VDDM_LVSupHiCFS_flg]
  [VPMM_PowerSta_enum] -> LV analog input error/2(VPMM_PowerSta_enum)
  LV analog input error/2(VDDM_LVInErrCFS_flg) -> [VDDM_LVInErrCFS_flg]
  [VDDM_AuxBattVolV_V] -> LV analog input error/6(VDDM_AuxBattVolV_V)
  [VINP_LVBattDet12V_V] -> LV analog input error/3(VINP_LVBattDet12V_V)
  [task_time_s] -> LV analog input error/1(task_time_s)
  [DTC_clear_request] -> LV analog input error/5(DTC_clear_request)
  [VINP_CANMsgValidBMS5_flg] -> LV analog input error/4(VINP_CANMsgValidBMS5_flg)
  LV analog input error/1(VDDM_LVInErrDTC_raw32) -> VDDM_LVInErrDTC_raw32/1
  [VDDM_IniLVLoCFS_flg] -> VDDM_IniLVLoCFS_flg/1
  [VDDM_LVSupLoCFS_flg] -> VDDM_LVSupLoCFS_flg/1
  [VDDM_LVSupHiCFS_flg] -> VDDM_LVSupHiCFS_flg/1
  [VDDM_LVInErrCFS_flg] -> VDDM_LVInErrCFS_flg/1
  VDDM_AuxBattVolV_V/1 -> [VDDM_AuxBattVolV_V]
  [VDDM_IniLVLoCFS_flg] -> Logical Operator/1
  [VDDM_LVSupLoCFS_flg] -> Logical Operator/2
  [VDDM_LVSupHiCFS_flg] -> Logical Operator/3
  [VDDM_LVInErrCFS_flg] -> Logical Operator/4
  Logical Operator/1 -> VDDM_PMMBattErr_flg/1  "VDDM_PMMBattErr_flg"
  VDDM_ClearZevDTCcmd_flg/1 -> [VDDM_ClearZevDTCcmd_flg]
  [VDDM_LVSupLoCFS_flg] -> Logical Operator1/1
  [VDDM_LVSupHiCFS_flg] -> Logical Operator1/2
  Logical Operator1/1 -> VDDM_EDriveSysErrLVSup_flg/1  "VDDM_EDriveSysErrLVSup_flg"
  Switch/1 -> [VDDM_AuxBatVolt_V]  "VDDM_AuxBatVolt_V"
  [VINP_VehicleType_enum] -> Relational Operator5/1
  [VINP_LVBattDet12V_V] -> Switch/3
  Relational Operator5/1 -> Switch/2
  Constant7/1 -> Relational Operator5/2
  [VDDM_AuxBattVolV_V] -> Switch/1
  VINP_VehicleType_enum/1 -> [VINP_VehicleType_enum]
  [VINP_CANMsgValidBMS5_flg] -> Initial LV battery voltage too low/5(VINP_CANMsgValidBMS5_flg)
  [VPMM_PowerSta_enum] -> Initial LV battery voltage too low/2(VPMM_PowerSta_enum)
  Initial LV battery voltage too low/2(VDDM_IniLVLoCFS_flg) -> [VDDM_IniLVLoCFS_flg]
  [VDDM_AuxBatVolt_V] -> Initial LV battery voltage too low/4(VDDM_AuxBatVolt_V)
  Initial LV battery voltage too low/1(VDDM_IniLVLoDTC_raw32) -> VDDM_IniLVLoDTC_raw32/1  "VDDM_IniLVLoDTC_raw32"
  [VDDM_ClearZevDTCcmd_flg] -> Initial LV battery voltage too low/6(DTC_clear_request)
  [task_time_s] -> Initial LV battery voltage too low/1(task_time_s)
  [VPMM_PwrStaSW_enum] -> Initial LV battery voltage too low/3(VPMM_PwrStaSW_enum)
  Switch2/1 -> [VINP_CANMsgValidBMS5_flg]
  Constant1/1 -> Relational Operator1/2
  Relational Operator1/1 -> Switch2/2
  [VINP_VehicleType_enum] -> Relational Operator1/1
  VINP_CANMsgValidBMS5_flg/1 -> Switch2/3
  Constant2/1 -> Switch2/1
  [VINP_VehicleType_enum] -> LV analog input error/7(VINP_VehicleType_enum)

== system ddm/DDM/DDM/PMM/SW failure ==
  task_time_s : Inport
  VPMM_PwrStaSW_enum : Inport  Port=2
  VPMM_PowerSta_enum : Inport  Port=3
  DTC_clear_request : Inport  Port=4
  VINP_DrStSW : Inport  Port=5
  VINP_FLAJARSW : Inport  Port=6
  VINP_FRAJARSW : Inport  Port=7
  VINP_RLAJARSW : Inport  Port=8
  VINP_RRAJARSW : Inport  Port=9
  VINP_HoodSW : Inport  Port=10
  VINP_TailgaSW : Inport  Port=11
  VDDM_ClearZevDTCcmd_flg : Inport  Port=12
  Driver seat switch failure : Subsystem
  FL Door switch failure : Subsystem
  FR Door switch failure : Subsystem
  Hood switch failure : Subsystem
  Logical Operator14 : Logic  Operator=OR  Inputs=6  AllPortsSameDT=off  OutDataTypeStr=boolean
  RL Door switch failure : Subsystem
  RR Door switch failure : Subsystem
  Tailgate switch failure : Subsystem
  VDDM_DrStSWDTC_raw32 : Outport
  VDDM_FLDoorSWDTC_raw32 : Outport  Port=2
  VDDM_RLDoorSWDTC_raw32 : Outport  Port=3
  VDDM_FRDoorSWDTC_raw32 : Outport  Port=4
  VDDM_RRDoorSWDTC_raw32 : Outport  Port=5
  VDDM_HoodSWDTC_raw32 : Outport  Port=6
  VDDM_TailgaSWDTC_raw32 : Outport  Port=7
  VDDM_VCUFLDoorSta_flg : Outport  Port=8
  VDDM_VCUFRDoorSta_flg : Outport  Port=9
  VDDM_VCURLDoorSta_flg : Outport  Port=10
  VDDM_VCURRDoorSta_flg : Outport  Port=11
  VDDM_VCUHoodSWSta_flg : Outport  Port=12
  VDDM_VCUTailgateSWSta_flg : Outport  Port=13
  VDDM_DrStSWCFS_flg : Outport  Port=14
  VDDM_FLDoorSWCFS_flg : Outport  Port=15
  VDDM_RLDoorSWCFS_flg : Outport  Port=16
  VDDM_FRDoorSWCFS_flg : Outport  Port=17
  VDDM_RRDoorSWCFS_flg : Outport  Port=18
  VDDM_HoodSWCFS_flg : Outport  Port=19
  VDDM_TailgaSWCFS_flg : Outport  Port=20
  VDDM_4D2CErr_flg : Outport  Port=21
  wires:
  Tailgate switch failure/2(VDDM_VCUTailgateSWSta_flg) -> VDDM_VCUTailgateSWSta_flg/1
  Tailgate switch failure/1(VDDM_TailgaSWDTC_raw32) -> VDDM_TailgaSWDTC_raw32/1
  [VINP_TailgaSW] -> Tailgate switch failure/4(VINP_TailgaSW)
  [DTC_clear_request] -> Tailgate switch failure/5(DTC_clear_request)
  [VPMM_PwrStaSW_enum] -> Tailgate switch failure/3(VPMM_PwrStaSW_enum)
  [VPMM_PowerSta_enum] -> Tailgate switch failure/2(VPMM_PowerSta_enum)
  [task_time_s] -> Tailgate switch failure/1(task_time_s)
  Hood switch failure/2(VDDM_VCUHoodSWSta_flg) -> VDDM_VCUHoodSWSta_flg/1
  Hood switch failure/1(VDDM_HoodSWDTC_raw32) -> VDDM_HoodSWDTC_raw32/1
  [VDDM_ClearZevDTCcmd_flg] -> Hood switch failure/5(DTC_clear_request)
  [VINP_HoodSW] -> Hood switch failure/4(VINP_HoodSW)
  VINP_TailgaSW/1 -> [VINP_TailgaSW]
  VINP_HoodSW/1 -> [VINP_HoodSW]
  [VPMM_PwrStaSW_enum] -> Hood switch failure/3(VPMM_PwrStaSW_enum)
  [VPMM_PowerSta_enum] -> Hood switch failure/2(VPMM_PowerSta_enum)
  [task_time_s] -> Hood switch failure/1(task_time_s)
  RR Door switch failure/2(VDDM_VCURRDoorSta_flg) -> VDDM_VCURRDoorSta_flg/1
  RR Door switch failure/1(VDDM_RRDoorSWDTC_raw32) -> VDDM_RRDoorSWDTC_raw32/1
  [VDDM_ClearZevDTCcmd_flg] -> RR Door switch failure/5(DTC_clear_request)
  [VINP_RRAJARSW] -> RR Door switch failure/4(VINP_RRAJARSW)
  [VPMM_PwrStaSW_enum] -> RR Door switch failure/3(VPMM_PwrStaSW_enum)
  [VPMM_PowerSta_enum] -> RR Door switch failure/2(VPMM_PowerSta_enum)
  [task_time_s] -> RR Door switch failure/1(task_time_s)
  RL Door switch failure/2(VDDM_VCURLDoorSta_flg) -> VDDM_VCURLDoorSta_flg/1
  RL Door switch failure/1(VDDM_RLDoorSWDTC_raw32) -> VDDM_RLDoorSWDTC_raw32/1
  [VDDM_ClearZevDTCcmd_flg] -> RL Door switch failure/5(DTC_clear_request)
  [VINP_RLAJARSW] -> RL Door switch failure/4(VINP_RLAJARSW)
  [task_time_s] -> RL Door switch failure/1(task_time_s)
  [VPMM_PowerSta_enum] -> RL Door switch failure/2(VPMM_PowerSta_enum)
  [VPMM_PwrStaSW_enum] -> RL Door switch failure/3(VPMM_PwrStaSW_enum)
  FR Door switch failure/2(VDDM_VCUFRDoorSta_flg) -> VDDM_VCUFRDoorSta_flg/1
  FR Door switch failure/1(VDDM_FRDoorSWDTC_raw32) -> VDDM_FRDoorSWDTC_raw32/1
  [VDDM_ClearZevDTCcmd_flg] -> FR Door switch failure/5(DTC_clear_request)
  [VINP_FRAJARSW] -> FR Door switch failure/4(VINP_FRAJARSW)
  [VPMM_PwrStaSW_enum] -> FR Door switch failure/3(VPMM_PwrStaSW_enum)
  [VPMM_PowerSta_enum] -> FR Door switch failure/2(VPMM_PowerSta_enum)
  [task_time_s] -> FR Door switch failure/1(task_time_s)
  FL Door switch failure/2(VDDM_VCUFLDoorSta_flg) -> VDDM_VCUFLDoorSta_flg/1
  FL Door switch failure/1(VDDM_FLDoorSWDTC_raw32) -> VDDM_FLDoorSWDTC_raw32/1
  [VDDM_ClearZevDTCcmd_flg] -> FL Door switch failure/5(DTC_clear_request)
  [VINP_FLAJARSW] -> FL Door switch failure/4(VINP_FLAJARSW)
  [VPMM_PwrStaSW_enum] -> FL Door switch failure/3(VPMM_PwrStaSW_enum)
  [VPMM_PowerSta_enum] -> FL Door switch failure/2(VPMM_PowerSta_enum)
  [task_time_s] -> FL Door switch failure/1(task_time_s)
  VINP_RRAJARSW/1 -> [VINP_RRAJARSW]
  VINP_RLAJARSW/1 -> [VINP_RLAJARSW]
  VINP_FRAJARSW/1 -> [VINP_FRAJARSW]
  VINP_FLAJARSW/1 -> [VINP_FLAJARSW]
  Driver seat switch failure/2(VDDM_DrStSWCFS_flg) -> VDDM_DrStSWCFS_flg/1
  DTC_clear_request/1 -> [DTC_clear_request]
  VPMM_PowerSta_enum/1 -> [VPMM_PowerSta_enum]
  VPMM_PwrStaSW_enum/1 -> [VPMM_PwrStaSW_enum]
  task_time_s/1 -> [task_time_s]
  VINP_DrStSW/1 -> [VINP_DrStSW]
  [task_time_s] -> Driver seat switch failure/1(task_time_s)
  [VINP_DrStSW] -> Driver seat switch failure/4(VINP_DrStSW)
  [VDDM_ClearZevDTCcmd_flg] -> Driver seat switch failure/5(DTC_clear_request)
  [VPMM_PwrStaSW_enum] -> Driver seat switch failure/3(VPMM_PwrStaSW_enum)
  [VPMM_PowerSta_enum] -> Driver seat switch failure/2(VPMM_PowerSta_enum)
  Driver seat switch failure/1(VDDM_DrStSWDTC_raw32) -> VDDM_DrStSWDTC_raw32/1
  FL Door switch failure/3(VDDM_FLDoorSWCFS_flg) -> [VDDM_FLDoorSWCFS_flg], VDDM_FLDoorSWCFS_flg/1
  RL Door switch failure/3(VDDM_RLDoorSWCFS_flg) -> [VDDM_RLDoorSWCFS_flg], VDDM_RLDoorSWCFS_flg/1
  FR Door switch failure/3(VDDM_FRDoorSWCFS_flg) -> [VDDM_FRDoorSWCFS_flg], VDDM_FRDoorSWCFS_flg/1
  RR Door switch failure/3(VDDM_RRDoorSWCFS_flg) -> [VDDM_RRDoorSWCFS_flg], VDDM_RRDoorSWCFS_flg/1
  Hood switch failure/3(VDDM_HoodSWCFS_flg) -> [VDDM_HoodSWCFS_flg], VDDM_HoodSWCFS_flg/1
  Tailgate switch failure/3(VDDM_TailgaSWCFS_flg) -> [VDDM_TailgaSWCFS_flg], VDDM_TailgaSWCFS_flg/1
  VDDM_ClearZevDTCcmd_flg/1 -> [VDDM_ClearZevDTCcmd_flg]
  [VDDM_RLDoorSWCFS_flg] -> Logical Operator14/3
  [VDDM_TailgaSWCFS_flg] -> Logical Operator14/6
  [VDDM_FLDoorSWCFS_flg] -> Logical Operator14/1
  [VDDM_HoodSWCFS_flg] -> Logical Operator14/5
  [VDDM_RRDoorSWCFS_flg] -> Logical Operator14/4
  [VDDM_FRDoorSWCFS_flg] -> Logical Operator14/2
  Logical Operator14/1 -> [VDDM_4D2CErr_flg]  "VDDM_4D2CErr_flg"
  [VDDM_4D2CErr_flg] -> VDDM_4D2CErr_flg/1

== system ddm/DDM/DDM/PMM/System conditions of ON to READY not satisfied ==
  note: Release Condition After Decision
  note: Test Detection Criteria
  note: Diagnostics and Fault Handling
  note: Test Pass Criteria
  task_time_s : Inport
  VPMM_PowerSta_enum : Inport  Port=2
  VPMM_PwrStaSW_enum : Inport  Port=3
  DTC_clear_request : Inport  Port=4
  VPMM_MCUReady_flg : Inport  Port=5
  VINP_AllowMovThd_OTA_enum : Inport  Port=6
  VDDM_KeyAuthCFS_flg : Inport  Port=7
  VDDM_FLDoorSWCFS_flg : Inport  Port=8
  VDDM_RLDoorSWCFS_flg : Inport  Port=9
  VDDM_FRDoorSWCFS_flg : Inport  Port=10
  VDDM_RRDoorSWCFS_flg : Inport  Port=11
  VDDM_HoodSWCFS_flg : Inport  Port=12
  VDDM_TailgaSWCFS_flg : Inport  Port=13
  Constant{1..2,12,22} (4 alike) : Constant  Value=FALSE
  Constant10 : Constant  Value=ENUM_POWERSTA_STANDBY
  Constant13 : Constant  Value=KDDM_ONtoRdyPassTO_s
  Constant14 : Constant  Value=KDDM_ONtoRdyPassTO_s
  Constant17 : Constant  Value=KDDM_ONtoRdyDetTO_s
  Constant18 : Constant  Value=KDDM_ONtoRdyDTC_cnt
  Constant28 : Constant  Value=ENUM_PWRSTASW_ON
  Constant29 : Constant  Value=ENUM_PWRSTASW_ON
  Constant3 : Constant  Value=TRUE
  Constant30 : Constant  Value=KDDM_ONtoRdyDiagnosisOffSW_flg
  Constant31 : Constant  Value=ENUM_POWERSTA_OFF
  Constant32 : Constant  Value=ENUM_ALLOWMOV_ALLOWREADY
  Constant34 : Constant  Value=ZERO_INT
  Constant35 : Constant  Value=KDDM_ONtoRdyDTC_cnt
  Constant4 : Constant  Value=TRUE
  Constant5 : Constant  Value=ENUM_ALLOWMOV_ALLOWREADY
  Constant6 : Constant  Value=TRUE
  DTC_Couter1 : hcu_lib/Basic_Blocks/DTC_Couter
  DTC_Info : hcu_lib/Basic_Blocks/DTC_Info
  Equal1 : RelationalOperator  Operator=~=  OutDataTypeStr=boolean  RndMeth=Simplest
  Equal{8,10,12,14} (4 alike) : RelationalOperator  Operator===  OutDataTypeStr=boolean  RndMeth=Simplest
  Equal11 : RelationalOperator  Operator=~=  OutDataTypeStr=boolean  RndMeth=Simplest
  Equal13 : RelationalOperator  OutDataTypeStr=boolean  RndMeth=Simplest
  Logical Operator1 : Logic  Operator=NOT  AllPortsSameDT=off  OutDataTypeStr=boolean
  Logical Operator14 : Logic  Operator=NOT  AllPortsSameDT=off  OutDataTypeStr=boolean
  Logical Operator16 : Logic  Operator=OR  Inputs=4  AllPortsSameDT=off  OutDataTypeStr=boolean
  Logical Operator17 : Logic  AllPortsSameDT=off  OutDataTypeStr=boolean
  Logical Operator2 : Logic  Operator=OR  Inputs=9  AllPortsSameDT=off  OutDataTypeStr=boolean
  Logical Operator20 : Logic  Operator=OR  Inputs=9  AllPortsSameDT=off  OutDataTypeStr=boolean
  Logical Operator21 : Logic  Operator=NOT  AllPortsSameDT=off  OutDataTypeStr=boolean
  Relational Operator1 : RelationalOperator  Operator=>  OutDataTypeStr=boolean  RndMeth=Simplest
  Switch{1..4,9} (5 alike) : Switch  Criteria=u2 ~= 0
  Terminator : Terminator
  Test Detection Criteria1 : hcu_lib/Basic_Blocks/Test Detection Criteria
  Timer2 : hcu_lib/Basic_Blocks/Timer
  Unit Delay1 : UnitDelay  SampleTime=-1  HasFrameUpgradeWarning=on
  VDDM_ONtoRdyDTC_raw32 : Outport
  VDDM_ONtoRdyCFS_flg : Outport  Port=2
  VDDM_EDriveSysErrONtoRdy_flg : Outport  Port=3
  VDDM_SysAllowReadySta_flg : Outport  Port=4
  wires:
  [VDDM_RRDoorSWCFS_flg] -> Logical Operator2/7
  Logical Operator2/1 -> Switch3/1
  [VDDM_FRDoorSWCFS_flg] -> Logical Operator2/6
  [VDDM_RLDoorSWCFS_flg] -> Logical Operator2/5
  [VDDM_FLDoorSWCFS_flg] -> Logical Operator2/4
  [VPMM_MCUReady_flg] -> Logical Operator1/1
  [VDDM_TailgaSWCFS_flg] -> Logical Operator2/9
  [VDDM_HoodSWCFS_flg] -> Logical Operator2/8
  [VDDM_KeyAuthCFS_flg] -> Logical Operator2/3
  Equal1/1 -> Logical Operator2/2
  Constant5/1 -> Equal1/2
  [VINP_AllowMovThd_OTA_enum] -> Equal1/1
  Logical Operator1/1 -> Logical Operator2/1
  [VDDM_TailgaSWCFS_flg] -> Logical Operator20/9
  [VDDM_HoodSWCFS_flg] -> Logical Operator20/8
  [VDDM_RRDoorSWCFS_flg] -> Logical Operator20/7
  [VDDM_FRDoorSWCFS_flg] -> Logical Operator20/6
  [VDDM_RLDoorSWCFS_flg] -> Logical Operator20/5
  [VDDM_FLDoorSWCFS_flg] -> Logical Operator20/4
  VDDM_TailgaSWCFS_flg/1 -> [VDDM_TailgaSWCFS_flg]
  VDDM_HoodSWCFS_flg/1 -> [VDDM_HoodSWCFS_flg]
  VDDM_RRDoorSWCFS_flg/1 -> [VDDM_RRDoorSWCFS_flg]
  VDDM_FRDoorSWCFS_flg/1 -> [VDDM_FRDoorSWCFS_flg]
  VDDM_RLDoorSWCFS_flg/1 -> [VDDM_RLDoorSWCFS_flg]
  VDDM_FLDoorSWCFS_flg/1 -> [VDDM_FLDoorSWCFS_flg]
  Switch4/1 -> VDDM_SysAllowReadySta_flg/1  "VDDM_SysAllowReadySta_flg"
  Constant1/1 -> Switch4/3
  Constant4/1 -> Switch4/1
  [VDDM_ONtoRdyCFS_flg] -> Switch4/2
  Switch2/1 -> VDDM_EDriveSysErrONtoRdy_flg/1  "VDDM_EDriveSysErrONtoRdy_flg"
  Constant3/1 -> Switch2/1
  Constant2/1 -> Switch2/3
  [VDDM_ONtoRdyCFS_flg] -> Switch2/2
  [VDDM_ONtoRdyCFS_flg] -> VDDM_ONtoRdyCFS_flg/1
  [VPMM_PwrStaSW_enum] -> Equal12/1
  Constant29/1 -> Equal12/2
  Constant6/1 -> Switch3/3
  Equal12/1 -> Switch3/2
  Constant32/1 -> Equal11/2
  [VDDM_KeyAuthCFS_flg] -> Logical Operator20/3
  Equal11/1 -> Logical Operator20/2
  Logical Operator14/1 -> Logical Operator20/1
  [VPMM_MCUReady_flg] -> Logical Operator14/1
  [VINP_AllowMovThd_OTA_enum] -> Equal11/1
  Logical Operator16/1 -> [VDDM_ONtoRdyCFSRls_flg]  "VDDM_ONtoRdyCFSRls_flg"
  [VDDM_ONtoRdyCFSRls_flg] -> DTC_Couter1/2
  [VDDM_ONtoRdyDet_flg] -> DTC_Couter1/1
  DTC_Couter1/1 -> [VDDM_ONtoRdyCFS_flg]  "VDDM_ONtoRdyCFS_flg"
  Constant14/1 -> Equal13/2
  [VDDM_ONtoRdyCFSRls_flg] -> Switch9/2
  Unit Delay1/1 -> Equal14/1
  Relational Operator1/1 -> Terminator/1  "VDDM_ONtoRdyDFS_flg"
  Constant34/1 -> Relational Operator1/2
  [VPMM_PowerSta_enum] -> Unit Delay1/1
  Equal14/1 -> Logical Operator17/1
  Switch3/1 -> Logical Operator21/1, Timer2/2
  Constant30/1 -> Logical Operator16/4
  Switch9/1 -> Test Detection Criteria1/1
  [task_time_s] -> Test Detection Criteria1/2
  [task_time_s] -> Timer2/3
  Switch1/1 -> Switch9/3
  Logical Operator21/1 -> Timer2/1
  Logical Operator17/1 -> Logical Operator16/1
  Constant12/1 -> Switch1/3
  Equal10/1 -> Logical Operator17/2
  Constant31/1 -> Equal14/2
  [DTC_clear_request] -> Logical Operator16/2
  DTC_Couter1/2 -> Relational Operator1/1  "VDDM_ONtoRdyDTC_cnt"
  Logical Operator20/1 -> Switch1/1
  [VPMM_PowerSta_enum] -> Equal10/1
  Constant22/1 -> Switch9/1
  Timer2/1 -> Equal13/1
  Constant10/1 -> Equal10/2
  Test Detection Criteria1/1 -> [VDDM_ONtoRdyDet_flg]  "VDDM_ONtoRdyDet_flg"
  Equal8/1 -> Switch1/2
  Constant13/1 -> Timer2/4
  Constant18/1 -> Test Detection Criteria1/3
  Constant35/1 -> DTC_Couter1/3
  [VPMM_PwrStaSW_enum] -> Equal8/1
  Equal13/1 -> [VDDM_ONtoRdyPass_flg]  "VDDM_ONtoRdyPass_flg"
  Constant28/1 -> Equal8/2
  Constant17/1 -> Test Detection Criteria1/4
  [VDDM_ONtoRdyPass_flg] -> Logical Operator16/3
  DTC_clear_request/1 -> [DTC_clear_request]
  task_time_s/1 -> [task_time_s]
  VPMM_PwrStaSW_enum/1 -> [VPMM_PwrStaSW_enum]
  VPMM_PowerSta_enum/1 -> [VPMM_PowerSta_enum]
  VPMM_MCUReady_flg/1 -> [VPMM_MCUReady_flg]
  VINP_AllowMovThd_OTA_enum/1 -> [VINP_AllowMovThd_OTA_enum]
  DTC_Info/1 -> VDDM_ONtoRdyDTC_raw32/1  "VDDM_ONtoRdyDTC_raw32"
  [VDDM_ONtoRdyPass_flg] -> DTC_Info/2
  [VDDM_ONtoRdyCFS_flg] -> DTC_Info/3
  VDDM_KeyAuthCFS_flg/1 -> [VDDM_KeyAuthCFS_flg]
  [VDDM_ONtoRdyDet_flg] -> DTC_Info/1
  [DTC_clear_request] -> DTC_Info/4
